simulink model "simul3_1"  (R2021b)
settings: Solver=VariableStepAuto  StartTime=0.0  StopTime=10.0  RelTol=1e-3
settings Model: Creator=radek  LastModifiedBy=radek

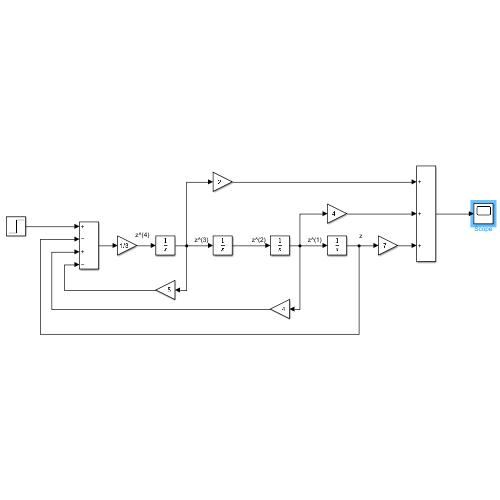
[thumbnail: Simulink's stored preview of the top-level diagram]
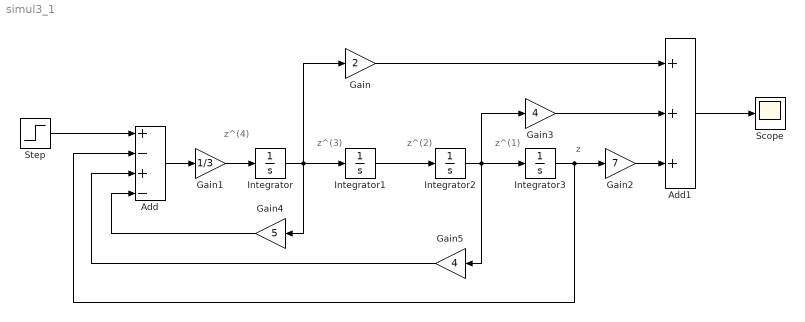
== system simul3_1 ==
  note: z
  note: z^(1)
  note: z^(2)
  note: z^(3)
  note: z^(4)
  Add : Sum  Inputs=+-+-
  Add1 : Sum  Inputs=+++
  Gain : Gain  Gain=2
  Gain1 : Gain  Gain=1/3
  Gain2 : Gain  Gain=7
  Gain3 : Gain  Gain=4
  Gain4 : Gain  Gain=5
  Gain5 : Gain  Gain=4
  Integrator{,1..3} (4 alike) : Integrator
  Scope : Scope
  Step : Step  SampleTime=0
  wires:
  Integrator/1 -> Integrator1/1, Gain/1, Gain4/1
  Integrator2/1 -> Gain5/1, Integrator3/1, Gain3/1
  Integrator3/1 -> Add/2, Gain2/1
  Gain/1 -> Add1/1
  Integrator1/1 -> Integrator2/1
  Gain2/1 -> Add1/3
  Gain3/1 -> Add1/2
  Add1/1 -> Scope/1
  Gain4/1 -> Add/4
  Gain5/1 -> Add/3
  Add/1 -> Gain1/1
  Step/1 -> Add/1
  Gain1/1 -> Integrator/1
